simulink model "Systems_Control"  (R2018a)
settings: Solver=ode45  StartTime=0.0  StopTime=500  RelTol=1e-6  EnableMultiTasking=on
values from neighbouring files (symbols this model uses):
  A = stateSpaceModel.A    [System_Control.m]    (also in script2.m)
  B = stateSpaceModel.B    [System_Control.m]    (also in script2.m)
  C = stateSpaceModel.C    [System_Control.m]    (also in script2.m)
  Nbar = Nu+K*Nx    [System_Control.m]    (also in script2.m)
  Ts = stateSpaceModel.Ts    [System_Control.m]    (also in script2.m)
undefined symbols (not defined in the file or in its folder): Atrue, Btrue, Ctrue, Dtrue, K, M
libraries: simulink x1
settings Model: Creator=jomle  LastModifiedBy=Gil
settings DataIOCC: LimitDataPoints=on  SaveFormat=Array
settings OptimizationCC: LifeSpan=inf
settings DebuggingCC: SFUnexpectedBacktrackingDiag=warning  SFNoUnconditionalDefaultTransitionDiag=warning  SFExecutionAtInitializationDiag=none
settings HardwareCC: ProdBitPerPointer=32  ProdBitPerSizeT=32  ProdBitPerPtrDiffT=32  ProdLargestAtomicFloat=None  ProdIntDivRoundTo=Undefined  ProdEndianess=Unspecified  ProdWordSize=32  ProdHWDeviceType=32-bit Generic
settings ModelReferenceCC: PropagateSignalLabelsOutOfModel=off
settings CodeAppCC: StateflowObjectComments=on
settings GRTTargetCC: TargetLangStandard=C89/C90 (ANSI)
settings ConfigComp: CovMetricSettings=dw  CovHtmlReporting=on  CovSaveCumulativeToWorkspaceVar=on  CovSaveSingleToWorkspaceVar=on  CovExternalEMLEnable=off

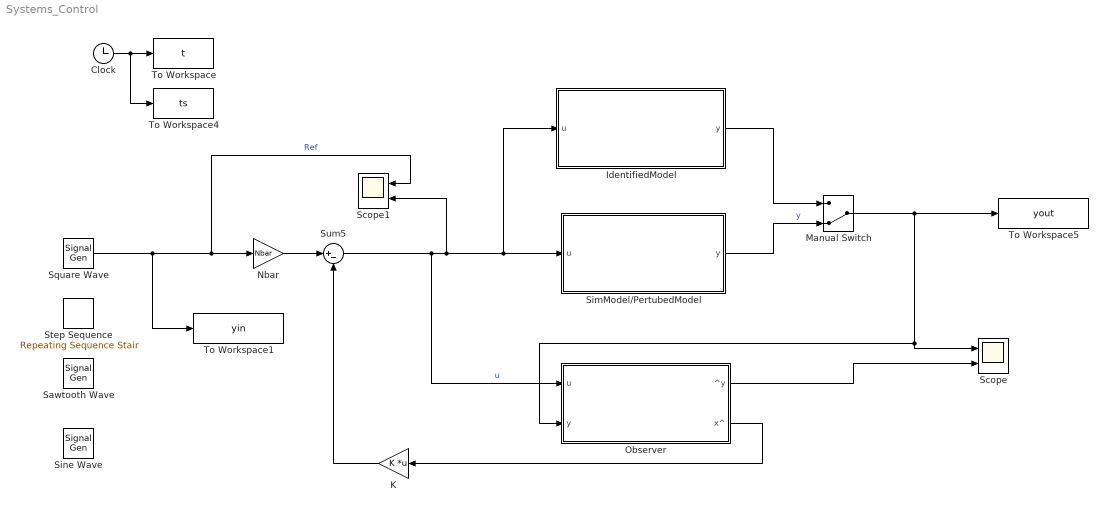
== system Systems_Control ==
  Clock : Clock
  IdentifiedModel : Subsystem
  K : Gain  Gain=K  Multiplication=Matrix(K*u)
  Manual Switch : ManualSwitch  CurrentSetting=0
  Nbar : Gain  Gain=Nbar
  Observer : Subsystem  Tag=Observer  Description=Observer
  Sawtooth Wave : SignalGenerator  WaveForm=square  Amplitude=4  Frequency=1/50
  Scope : Scope  NumInputPorts=2
  Scope1 : Scope  NumInputPorts=2
  SimModel/PertubedModel : Subsystem
  Sine Wave : SignalGenerator  Amplitude=4  Frequency=1/50
  Square Wave : SignalGenerator  WaveForm=square  Amplitude=4  Frequency=1/50
  Step Sequence : simulink/Sources/Repeating Sequence Stair  OutValues=[1 4 2 3].'  tsamp=20  OutMin=[]  OutMax=[]  OutDataTypeStr=double  OutputDataTypeScalingMode=double  OutDataType=fixdt(0,8)  ConRadixGroup=Best Precision: Vector-wise  OutScaling=2^-12
  Sum5 : Sum  Inputs=|+-
  To Workspace : ToWorkspace  VariableName=t  SampleTime=-1
  To Workspace1 : ToWorkspace  VariableName=yin  SaveFormat=Structure With Time  SampleTime=Ts
  To Workspace4 : ToWorkspace  VariableName=ts  SampleTime=Ts
  To Workspace5 : ToWorkspace  VariableName=yout  SaveFormat=Structure With Time  SampleTime=Ts
  wires:
  Clock/1 -> To Workspace4/1, To Workspace/1
  Sum5/1 -> Observer/1(u), Scope1/2, IdentifiedModel/1(u), SimModel/PertubedModel/1(u)  "u"
  Nbar/1 -> Sum5/1
  K/1 -> Sum5/2
  Square Wave/1 -> To Workspace1/1, Scope1/1, Nbar/1  "Ref"
  Observer/1(^y) -> Scope/2
  Observer/2(x^) -> K/1
  Manual Switch/1 -> Scope/1, Observer/2(y), To Workspace5/1
  IdentifiedModel/1(y) -> Manual Switch/1
  SimModel/PertubedModel/1(y) -> Manual Switch/2  "y"

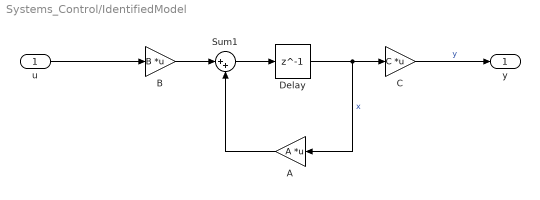
== system Systems_Control/IdentifiedModel ==
  u : Inport
  "A " : Gain  Gain=A  Multiplication=Matrix(K*u)
  B : Gain  Gain=B  Multiplication=Matrix(K*u)
  C : Gain  Gain=C  Multiplication=Matrix(K*u)
  Delay : Delay  DelayLength=1  InitialCondition=0  SampleTime=Ts
  Sum1 : Sum  Inputs=|++
  y : Outport
  wires:
  u/1 -> B/1
  "A "/1 -> Sum1/2
  B/1 -> Sum1/1
  Delay/1 -> "A "/1, C/1  "x"
  Sum1/1 -> Delay/1
  C/1 -> y/1  "y"

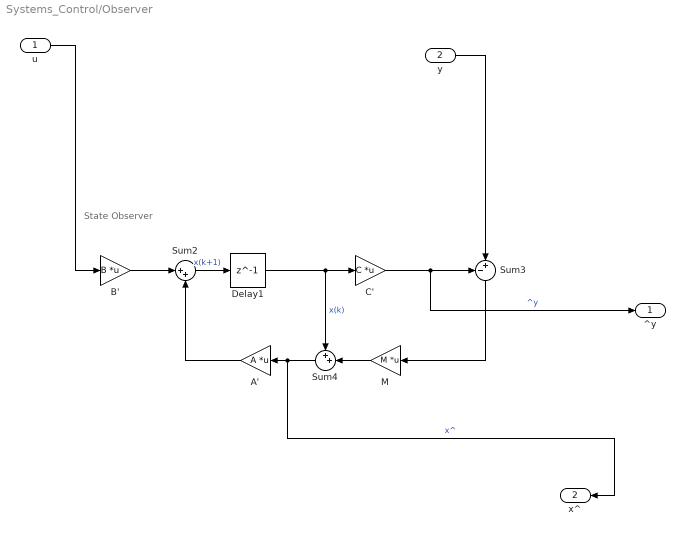
== system Systems_Control/Observer ==
  note: State Observer
  u : Inport
  y : Inport  Port=2
  A' : Gain  Gain=A  Multiplication=Matrix(K*u)
  B' : Gain  Gain=B  Multiplication=Matrix(K*u)
  C' : Gain  Gain=C  Multiplication=Matrix(K*u)
  Delay1 : Delay  DelayLength=1  InitialCondition=0  SampleTime=Ts
  M : Gain  Gain=M  Multiplication=Matrix(K*u)
  Sum2 : Sum  Inputs=|++
  Sum3 : Sum  Inputs=-+|
  Sum4 : Sum  Inputs=++|
  ^y : Outport
  x^ : Outport  Port=2
  wires:
  M/1 -> Sum4/2
  Sum3/1 -> M/1
  Sum4/1 -> x^/1, A'/1  "x^"
  y/1 -> Sum3/2
  C'/1 -> ^y/1, Sum3/1  "^y"
  A'/1 -> Sum2/2
  Delay1/1 -> Sum4/1, C'/1  "x(k)"
  B'/1 -> Sum2/1
  Sum2/1 -> Delay1/1  "x(k+1)"
  u/1 -> B'/1

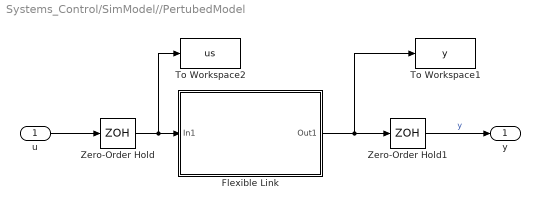
== system Systems_Control/SimModel//PertubedModel ==
  u : Inport
  Flexible Link : Subsystem
      mask Display: image('quanserlink.jpg')
  To Workspace1 : ToWorkspace  VariableName=y  SampleTime=-1
  To Workspace2 : ToWorkspace  VariableName=us  SampleTime=Ts
  Zero-Order Hold : ZeroOrderHold  SampleTime=Ts
  Zero-Order Hold1 : ZeroOrderHold  SampleTime=Ts
  y : Outport
  wires:
  Flexible Link/1(Out1) -> To Workspace1/1, Zero-Order Hold1/1
  Zero-Order Hold/1 -> To Workspace2/1, Flexible Link/1(In1)
  Zero-Order Hold1/1 -> y/1  "y"
  u/1 -> Zero-Order Hold/1

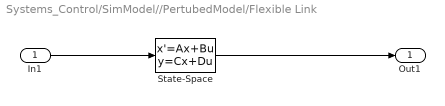
== system Systems_Control/SimModel//PertubedModel/Flexible Link ==
  In1 : Inport
  State-Space : StateSpace  A=Atrue  B=Btrue  C=Ctrue  D=Dtrue  InitialCondition=0
  Out1 : Outport
  wires:
  State-Space/1 -> Out1/1
  In1/1 -> State-Space/1
